simulink model "modeloSimulinkSimscapeHisteresisDeadTime"  (R2025b)
settings: Solver=FixedStepAuto  StartTime=0.0  StopTime=0.04  FixedStep=1e-7  RelTol=1e-3
undefined symbols (not defined in the file): alpha
libraries: fl_lib x50, nesl_utility x26, ee_lib x12, spsTriangleGeneratorLib x6
settings Model: Creator=rkhga  LastModifiedBy=daniel
settings SolverCC: EnableFixedStepZeroCrossing=on

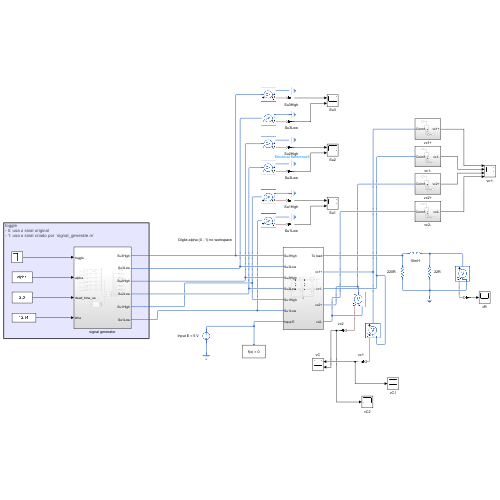
[thumbnail: Simulink's stored preview of the top-level diagram]
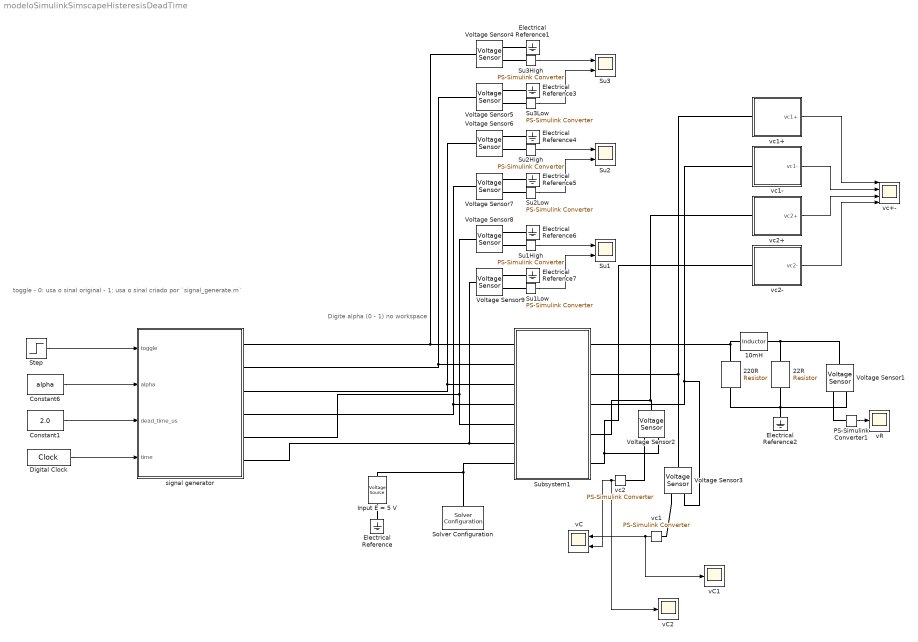
== system modeloSimulinkSimscapeHisteresisDeadTime ==
  note: toggle
      | - 0: usa o sinal original
      | - 1: usa o sinal criado por `signal_generate.m`
  note: Digite alpha (0 - 1) no workspace
  10mH : ee_lib/Passive/Inductor  l=10e-3 H  enable_L_tol=ee.enum.toleranceApplication.none  L_tol=20  tol_distribution=ee.enum.toleranceDistribution.uniform  nSigma=4  r=0 Ohm  g=1e-9 1/Ohm  enable_operating_limits=ee.enum.enable.no  operating_limit_action=ee.enum.passive.reportOpLim.warn  max_working_current=1 A  power_rating=1 W  i_L_specify=off  i_L_priority=High  i_L=0 A  i_L_nominal_specify=off  i_L_nominal_value=1  i_L_nominal_unit=A
  220R : ee_lib/Passive/Resistor  R=220 Ohm  enable_R_tol=ee.enum.toleranceApplication.none  R_tol=5  tol_distribution=ee.enum.toleranceDistribution.uniform  nSigma=4  enable_operating_limits=ee.enum.enable.no  operating_limit_action=ee.enum.passive.reportOpLim.warn  power_rating=1 W  max_working_voltage=100 V  noise_mode=ee.enum.sources.noise.Disabled  Tdevice=25 degC  sample_time=1e-3 s  repeatability=ee.enum.ic.repeatability.notRepeatable  user_seed=0  auto_seed=418932850  power_derating_T1=70 degC  power_derating_T2=155 degC  operating_temperature_range_vec=[-50, 150] degC  alpha=3.93e-3 1/K  Tmeas=25 degC  thermal_mass=100 J/K  temperature_specify=off  temperature_priority=High  temperature=298.15 K  temperature_nominal_specify=off  temperature_nominal_value=1  temperature_nominal_unit=K
  22R : ee_lib/Passive/Resistor  R=22 Ohm  enable_R_tol=ee.enum.toleranceApplication.none  R_tol=5  tol_distribution=ee.enum.toleranceDistribution.uniform  nSigma=4  enable_operating_limits=ee.enum.enable.no  operating_limit_action=ee.enum.passive.reportOpLim.warn  power_rating=1 W  max_working_voltage=100 V  noise_mode=ee.enum.sources.noise.Disabled  Tdevice=25 degC  sample_time=1e-3 s  repeatability=ee.enum.ic.repeatability.notRepeatable  user_seed=0  auto_seed=3890346746  power_derating_T1=70 degC  power_derating_T2=155 degC  operating_temperature_range_vec=[-50, 150] degC  alpha=3.93e-3 1/K  Tmeas=25 degC  thermal_mass=100 J/K  temperature_specify=off  temperature_priority=High  temperature=298.15 K  temperature_nominal_specify=off  temperature_nominal_value=1  temperature_nominal_unit=K
  Constant1 : Constant  Value=2.0
  Constant6 : Constant  Value=alpha
  Digital Clock : DigitalClock  SampleTime=1e-7
  Electrical Reference{,1..7} (8 alike) : fl_lib/Electrical/Electrical Elements/Electrical Reference
  Input E = 5 V : ee_lib/Sources/Voltage Source  dc_voltage=5 V  ac_voltage=0 V  ac_shift=0 rad  ac_frequency=60 Hz  noise_mode=ee.enum.sources.noise.Disabled  PSD=0 V^2/Hz  sample_time=1e-3 s  repeatability=ee.enum.sources.repeatability.NotRepeatable  user_seed=0  auto_seed=3499211588  i_specify=off  i_priority=None  i=0 A  i_nominal_specify=off  i_nominal_value=1  i_nominal_unit=A  v_specify=off  v_priority=None  v=0 V  v_nominal_specify=off  v_nominal_value=1  v_nominal_unit=V
  PS-Simulink Converter1 : nesl_utility/PS-Simulink Converter  PhysicalDomain=network_engine_domain  SubClassName=ps_output  LeftPortType=input  RightPortType=output  PseudoPeriodic=off  Frequencies=[]  VectorFormat=inherit  Unit=inherit  AffineConversion=off
  Solver Configuration : nesl_utility/Solver Configuration  PhysicalDomain=network_engine_domain  SubClassName=solver  LeftPortType=input  RightPortType=generic  Tones=[]  Harmonics=[]  SimulateNoise=off  Profile=off  UseLocalSampling=off  EnableSwitchedLinearOptims=on  FrequencyDomain=off  UseCCode=off  RelTol=0.001  AbsTol=0.001  MinStep=1e-09  ToWorkspace=off  RevertToSquareIcSolve=off  NumHomotopyIterations=100  PhasorMode=off  PhasorModeNumHarmonics=1  ConsistencySolver=NEWTON_XTOL_AFTER_FTOL  IndexReductionMethod=DerivativeReplacement  DoDC=off  ResidualTolerance=1e-09  ConsistencyTolSource=GLOBAL  ConsistencyAbsTol=0.001  ConsistencyRelTol=0.001  ConsistencyTolFactor=0.001  UseLocalSolver=off  LocalSolverChoice=NE_TRAPEZOIDAL_ADVANCER  ResolveIndetEquations=on  FunctionEvalNumThread=1  LocalSolverSampleTime=0.000001  DoFixedCost=off  MaxNonlinIter=3  MaxModeIter=2  ComputeImpulses=off  ImpulseIterations=2  LinearAlgebra=auto  LinearAlgebraNumThread=0  EquationFormulation=NE_TIME_EF  DelaysMemoryBudget=1024  AutomaticFiltering=on  FilteringTimeConstant=0.001  PartitionStorageMethod=AS_NEEDED  PartitionMemoryBudget=1024  PartitionMethod=ROBUST  MultibodyUseLocalSolver=off  MultibodyLocalSolverChoice=ODE1  MultibodyLocalSolverSampleTime=0.001
  Step : Step  Time=0  Before=1  After=0  SampleTime=0
  Su1 : Scope  NumInputPorts=2
      settings: ActiveDisplayYMinimum=0.99850460772373162  ActiveDisplayYMaximum=1.0003414939639432  DataLoggingVariableName=ScopeData3
  Su1High : nesl_utility/PS-Simulink Converter  PhysicalDomain=network_engine_domain  SubClassName=ps_output  LeftPortType=input  RightPortType=output  PseudoPeriodic=off  Frequencies=[]  VectorFormat=inherit  Unit=inherit  AffineConversion=off
  Su1Low : nesl_utility/PS-Simulink Converter  PhysicalDomain=network_engine_domain  SubClassName=ps_output  LeftPortType=input  RightPortType=output  PseudoPeriodic=off  Frequencies=[]  VectorFormat=inherit  Unit=inherit  AffineConversion=off
  Su2 : Scope  NumInputPorts=2
      settings: ActiveDisplayYMinimum=-1.01553  ActiveDisplayYMaximum=1.07216  DataLoggingVariableName=ScopeData2
  Su2High : nesl_utility/PS-Simulink Converter  PhysicalDomain=network_engine_domain  SubClassName=ps_output  LeftPortType=input  RightPortType=output  PseudoPeriodic=off  Frequencies=[]  VectorFormat=inherit  Unit=inherit  AffineConversion=off
  Su2Low : nesl_utility/PS-Simulink Converter  PhysicalDomain=network_engine_domain  SubClassName=ps_output  LeftPortType=input  RightPortType=output  PseudoPeriodic=off  Frequencies=[]  VectorFormat=inherit  Unit=inherit  AffineConversion=off
  Su3 : Scope  NumInputPorts=2
      settings: ActiveDisplayYMinimum=-1.25  ActiveDisplayYMaximum=1.25
  Su3High : nesl_utility/PS-Simulink Converter  PhysicalDomain=network_engine_domain  SubClassName=ps_output  LeftPortType=input  RightPortType=output  PseudoPeriodic=off  Frequencies=[]  VectorFormat=inherit  Unit=inherit  AffineConversion=off
  Su3Low : nesl_utility/PS-Simulink Converter  PhysicalDomain=network_engine_domain  SubClassName=ps_output  LeftPortType=input  RightPortType=output  PseudoPeriodic=off  Frequencies=[]  VectorFormat=inherit  Unit=inherit  AffineConversion=off
  Subsystem1 : Subsystem
  Voltage Sensor{1..9} (9 alike) : fl_lib/Electrical/Electrical Sensors/Voltage Sensor
  signal generator : Subsystem
      settings: PortSchema="{\"entries\":[{\"content\":{\"sides\":[{\"content\":{\"connectorIds\":[\"LConn1\",\"LConn2\",\"LConn3\",\"LConn4\",\"LConn5\",\"LConn6\"]},\"type\":\"ConnectorPlacement.EquallySpacedRectSide\",\"uuid\":\"aa1a153a-1645-4c3d-b48e-03759f31f217\"},{\"content\":{\"connectorIds\":[\"In1\",\"In2\",\"In3\",\"In4\"],\"side\":\"RIGHT\"},\"type\":\"ConnectorPlacement.EquallySpacedRectSide\",\"uuid\":\"be438c4b-dc66-4eaf-bb53-25e90e68573c\"},{\"content\":{\"side\":\"TOP\"},\"type\":\"ConnectorPlacement.EquallySpacedRectSide\",\"uuid\":\"4362158f-9cc4-444f-8c13-d432f498cf5b\"}]},\"type\":\"ConnectorPlacement.EquallySpacedConnector\",\"uuid\":\"f810cfc3-0b98-45ae-8d35-8e9d04ff1bd5\"}],\"packageUris\":[\"http://schema.mathworks.com/mf0/Connector/R2020b\"],\"version\":\"1.0\"}"
  vC : Scope  NumInputPorts=2
      settings: ActiveDisplayYMinimum=-0.84659912811996252  ActiveDisplayYMaximum=6.9513683577501517
  vC1 : Scope
      settings: ActiveDisplayYMinimum=1.5127533601392706  ActiveDisplayYMaximum=1.8347191591870249  DataLoggingVariableName=ScopeData4
  vC2 : Scope
      settings: ActiveDisplayYMinimum=3.0808662411635424  ActiveDisplayYMaximum=3.5294915136441256  DataLoggingVariableName=ScopeData5
  vR : Scope
      settings: ActiveDisplayYMinimum=0.27238883407399678  ActiveDisplayYMaximum=0.38136658735243295
  vc+- : Scope  NumInputPorts=4
      settings: ActiveDisplayYMinimum=-18.52788  ActiveDisplayYMaximum=9.39765
  vc1 : nesl_utility/PS-Simulink Converter  PhysicalDomain=network_engine_domain  SubClassName=ps_output  LeftPortType=input  RightPortType=output  PseudoPeriodic=off  Frequencies=[]  VectorFormat=inherit  Unit=inherit  AffineConversion=off
  vc1+ : Subsystem
  vc1- : Subsystem
  vc2 : nesl_utility/PS-Simulink Converter  PhysicalDomain=network_engine_domain  SubClassName=ps_output  LeftPortType=input  RightPortType=output  PseudoPeriodic=off  Frequencies=[]  VectorFormat=inherit  Unit=inherit  AffineConversion=off
  vc2+ : Subsystem
  vc2- : Subsystem
  wires:
  PS-Simulink Converter1/1 -> vR/1
  vc1/1 -> vC1/1, vC/1
  Su3High/1 -> Su3/1
  Su3Low/1 -> Su3/2
  Su2High/1 -> Su2/1
  Su2Low/1 -> Su2/2
  Su1High/1 -> Su1/1
  Su1Low/1 -> Su1/2
  vc2/1 -> vC2/1, vC/2
  vc2+/1(vc2+) -> vc+-/3
  vc1-/1(vc1-) -> vc+-/2
  vc2-/1(vc2-) -> vc+-/4
  vc1+/1(vc1+) -> vc+-/1
  Step/1 -> signal generator/1(toggle)
  Constant6/1 -> signal generator/2(alpha)
  Digital Clock/1 -> signal generator/4(time)
  Constant1/1 -> signal generator/3(dead_time_us)
  connections:
  Electrical Reference/LConn1 -- Input E = 5 V/RConn1
  Subsystem1/LConn7 -- Solver Configuration/RConn1 -- Input E = 5 V/LConn1
  22R/RConn1 -- 220R/RConn1 -- Electrical Reference2/LConn1 -- Voltage Sensor1/RConn2
  Voltage Sensor1/LConn1 -- 10mH/RConn1 -- 22R/LConn1
  Voltage Sensor1/RConn1 -- PS-Simulink Converter1/LConn1
  220R/LConn1 -- 10mH/LConn1 -- Subsystem1/RConn1
  Subsystem1/LConn1 -- Voltage Sensor4/LConn1 -- signal generator/LConn1
  Subsystem1/LConn2 -- Voltage Sensor5/LConn1 -- signal generator/LConn2
  Subsystem1/LConn3 -- Voltage Sensor6/LConn1 -- signal generator/LConn3
  signal generator/LConn4 -- Voltage Sensor7/LConn1 -- Subsystem1/LConn4
  Subsystem1/LConn5 -- signal generator/LConn5 -- Voltage Sensor8/LConn1
  signal generator/LConn6 -- Voltage Sensor9/LConn1 -- Subsystem1/LConn6
  Subsystem1/RConn4 -- vc2+/LConn1 -- Voltage Sensor2/LConn1
  Voltage Sensor2/RConn2 -- vc2-/LConn1 -- Subsystem1/RConn5
  Voltage Sensor3/RConn1 -- vc1/LConn1
  Subsystem1/RConn2 -- vc1+/LConn1 -- Voltage Sensor3/LConn1
  Subsystem1/RConn3 -- vc1-/LConn1 -- Voltage Sensor3/RConn2
  Electrical Reference1/LConn1 -- Voltage Sensor4/RConn2
  Voltage Sensor5/RConn2 -- Electrical Reference3/LConn1
  Voltage Sensor4/RConn1 -- Su3High/LConn1
  Su3Low/LConn1 -- Voltage Sensor5/RConn1
  Voltage Sensor6/RConn1 -- Su2High/LConn1
  Electrical Reference4/LConn1 -- Voltage Sensor6/RConn2
  Su2Low/LConn1 -- Voltage Sensor7/RConn1
  Voltage Sensor7/RConn2 -- Electrical Reference5/LConn1
  Voltage Sensor8/RConn1 -- Su1High/LConn1
  Voltage Sensor9/RConn2 -- Electrical Reference7/LConn1
  Electrical Reference6/LConn1 -- Voltage Sensor8/RConn2
  Su1Low/LConn1 -- Voltage Sensor9/RConn1
  Voltage Sensor2/RConn1 -- vc2/LConn1

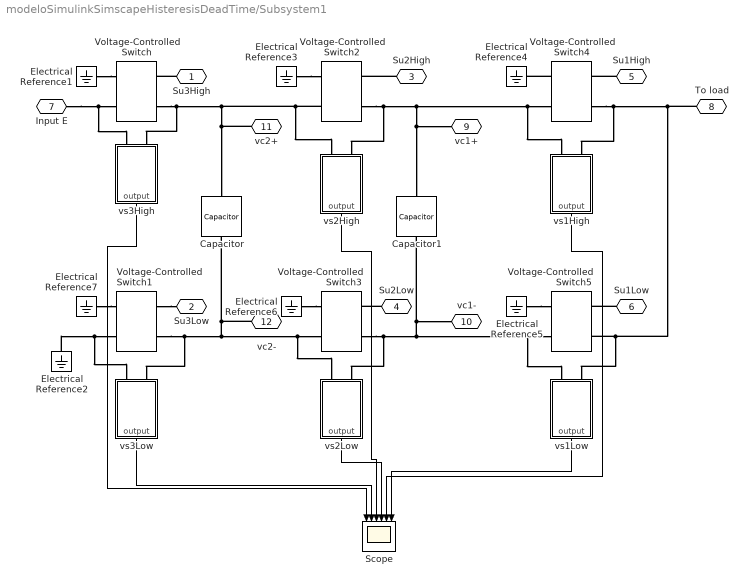
== system modeloSimulinkSimscapeHisteresisDeadTime/Subsystem1 ==
  Capacitor : ee_lib/Passive/Capacitor  cap_option=ee.enum.passive.capacitor.capOption.const  c=2.1e-6 F  Cvec=[1e-05, 1e-06] F  Vvec=[0, 10] V  CV_table_symmetry=ee.enum.passive.capacitor.tableSymmetry.yes  f_vec=[1, 10] kHz  DFext_vec=[.8, 1.2]  enable_C_tol=ee.enum.toleranceApplication.none  averaging_period=0 s  C_tol=5  tol_distribution=ee.enum.toleranceDistribution.uniform  nSigma=4  r=0 Ohm  g=0 1/Ohm  enable_operating_limits=ee.enum.enable.no  operating_limit_action=ee.enum.passive.reportOpLim.warn  max_working_voltage_range=[-25, 25] V  power_rating=1 W  maxTemperature=85 degC  thermalEnable=false  thermalMass=1 J/K  i_specify=off  i_priority=None  i=0 A  i_nominal_specify=off  i_nominal_value=1  i_nominal_unit=A  v_specify=off  v_priority=None  v=0 V  v_nominal_specify=off  v_nominal_value=1  v_nominal_unit=V  vc_specify=off  vc_priority=High  vc=0 V  vc_nominal_specify=off  vc_nominal_value=1  vc_nominal_unit=V  T_specify=off  T_priority=None  T=298.15 K  T_nominal_specify=off  T_nominal_value=1  T_nominal_unit=K
  Capacitor1 : ee_lib/Passive/Capacitor  cap_option=ee.enum.passive.capacitor.capOption.const  c=2.1e-6 F  Cvec=[1e-05, 1e-06] F  Vvec=[0, 10] V  CV_table_symmetry=ee.enum.passive.capacitor.tableSymmetry.yes  f_vec=[1, 10] kHz  DFext_vec=[.8, 1.2]  enable_C_tol=ee.enum.toleranceApplication.none  averaging_period=0 s  C_tol=5  tol_distribution=ee.enum.toleranceDistribution.uniform  nSigma=4  r=0 Ohm  g=0 1/Ohm  enable_operating_limits=ee.enum.enable.no  operating_limit_action=ee.enum.passive.reportOpLim.warn  max_working_voltage_range=[-25, 25] V  power_rating=1 W  maxTemperature=85 degC  thermalEnable=false  thermalMass=1 J/K  i_specify=off  i_priority=None  i=0 A  i_nominal_specify=off  i_nominal_value=1  i_nominal_unit=A  v_specify=off  v_priority=None  v=0 V  v_nominal_specify=off  v_nominal_value=1  v_nominal_unit=V  vc_specify=off  vc_priority=High  vc=0 V  vc_nominal_specify=off  vc_nominal_value=1  vc_nominal_unit=V  T_specify=off  T_priority=None  T=298.15 K  T_nominal_specify=off  T_nominal_value=1  T_nominal_unit=K
  Electrical Reference{1..7} (7 alike) : fl_lib/Electrical/Electrical Elements/Electrical Reference
  Scope : Scope  NumInputPorts=6
      settings: ActiveDisplayYMinimum=-8.8853464798149755  ActiveDisplayYMaximum=25.227625908816535  DataLoggingVariableName=ScopeData2
  Voltage-Controlled Switch{,1..5} (6 alike) : ee_lib/Additional Components/SPICE Passives/Voltage-Controlled Switch  SWITCH_model=ee.enum.switches.switchModelVoltage.transition  VON=1 V  VOFF=0 V  VT=0 V  VH=0 V  RON=1e-12 Ohm  ROFF_res=1e6 Ohm  Roff_gmin=ee.enum.switches.offResistance.no  ROFF=1e12 Ohm  TD=0 s
      settings: InternalSimscapePortConfiguration="{\"Bottom\":[],\"Left\":[{\"id\":\"p1\",\"label\":\"1+\",\"type\":\"foundation.electrical.electrical\"},{\"id\":\"p2\",\"label\":\"2+\",\"type\":\"foundation.electrical.electrical\"}],\"Right\":[{\"id\":\"n1\",\"label\":\"1-\",\"type\":\"foundation.electrical.electrical\"},{\"id\":\"n2\",\"label\":\"2-\",\"type\":\"foundation.electrical.electrical\"}],\"Top\":[]}"
  vs1High : Subsystem
  vs1Low : Subsystem
  vs2High : Subsystem
  vs2Low : Subsystem
  vs3High : Subsystem
  vs3Low : Subsystem
  Su3High : PMIOPort  Side=Left
  Su3Low : PMIOPort  Port=2  Side=Left
  Su2High : PMIOPort  Port=3  Side=Left
  Su2Low : PMIOPort  Port=4  Side=Left
  Su1High : PMIOPort  Port=5  Side=Left
  Su1Low : PMIOPort  Port=6  Side=Left
  Input E : PMIOPort  Port=7  Side=Left
  To load : PMIOPort  Port=8  Side=Right
  vc1+ : PMIOPort  Port=9  Side=Right
  vc1- : PMIOPort  Port=10  Side=Right
  vc2+ : PMIOPort  Port=11  Side=Right
  vc2- : PMIOPort  Port=12  Side=Right
  wires:
  vs2Low/1(output) -> Scope/4
  vs1Low/1(output) -> Scope/6
  vs3Low/1(output) -> Scope/2
  vs2High/1(output) -> Scope/3
  vs1High/1(output) -> Scope/5
  vs3High/1(output) -> Scope/1
  connections:
  Su2Low/RConn1 -- Voltage-Controlled Switch3/LConn1
  Voltage-Controlled Switch2/LConn2 -- vs2High/LConn2 -- vc1+/RConn1 -- Capacitor1/LConn1 -- vs1High/LConn1 -- Voltage-Controlled Switch4/RConn2
  Input E/RConn1 -- vs3High/LConn1 -- Voltage-Controlled Switch/RConn2
  Voltage-Controlled Switch/LConn2 -- vs2High/LConn1 -- Voltage-Controlled Switch2/RConn2 -- vc2+/RConn1 -- Capacitor/LConn1 -- vs3High/LConn2
  Voltage-Controlled Switch3/LConn2 -- vs2Low/LConn2 -- Capacitor1/RConn1 -- vc1-/RConn1 -- vs1Low/LConn1 -- Voltage-Controlled Switch5/RConn2
  Voltage-Controlled Switch1/LConn2 -- vs3Low/LConn2 -- Capacitor/RConn1 -- vc2-/RConn1 -- vs2Low/LConn1 -- Voltage-Controlled Switch3/RConn2
  Voltage-Controlled Switch4/LConn2 -- vs1High/LConn2 -- To load/RConn1 -- vs1Low/LConn2 -- Voltage-Controlled Switch5/LConn2
  Electrical Reference2/LConn1 -- vs3Low/LConn1 -- Voltage-Controlled Switch1/RConn2
  Voltage-Controlled Switch1/LConn1 -- Su3Low/RConn1
  Su1High/RConn1 -- Voltage-Controlled Switch4/LConn1
  Su2High/RConn1 -- Voltage-Controlled Switch2/LConn1
  Su3High/RConn1 -- Voltage-Controlled Switch/LConn1
  Electrical Reference1/LConn1 -- Voltage-Controlled Switch/RConn1
  Electrical Reference3/LConn1 -- Voltage-Controlled Switch2/RConn1
  Electrical Reference5/LConn1 -- Voltage-Controlled Switch5/RConn1
  Electrical Reference6/LConn1 -- Voltage-Controlled Switch3/RConn1
  Su1Low/RConn1 -- Voltage-Controlled Switch5/LConn1
  Electrical Reference7/LConn1 -- Voltage-Controlled Switch1/RConn1
  Voltage-Controlled Switch4/RConn1 -- Electrical Reference4/LConn1

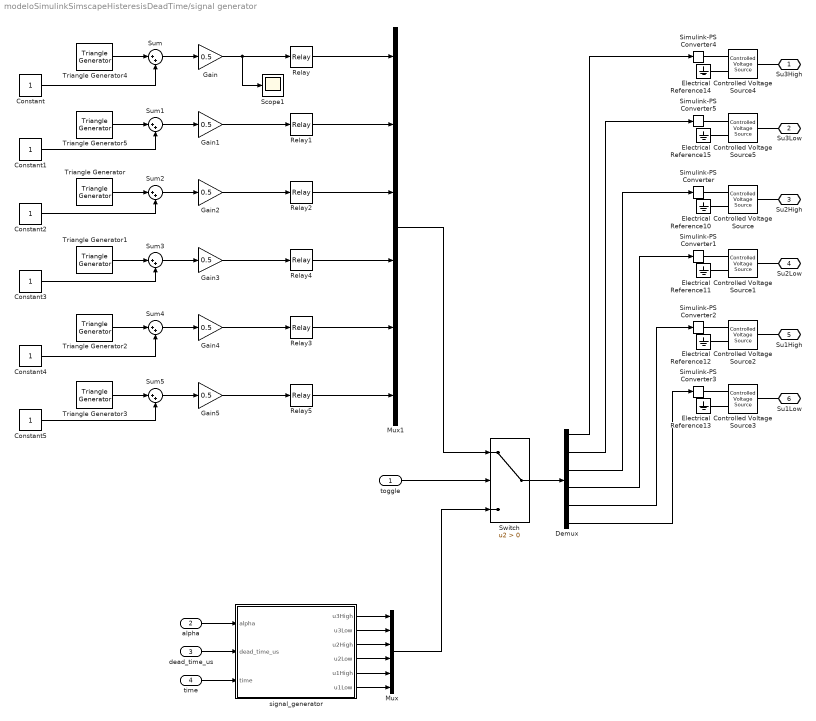
== system modeloSimulinkSimscapeHisteresisDeadTime/signal generator ==
  toggle : Inport
  alpha : Inport  Port=2
  dead_time_us : Inport  Port=3
  time : Inport  Port=4
  Constant{,1..5} (6 alike) : Constant
  Controlled Voltage Source{,1..5} (6 alike) : fl_lib/Electrical/Electrical Sources/Controlled Voltage Source
  Demux : Demux  Outputs=6
  Electrical Reference{10..15} (6 alike) : fl_lib/Electrical/Electrical Elements/Electrical Reference
  Gain{,1..5} (6 alike) : Gain  Gain=0.5
  Mux : Mux  Inputs=6
  Mux1 : Mux  Inputs=6
  Relay : Relay  OnSwitchValue=alpha  OffSwitchValue=alpha - 2/141  OnOutputValue=-1  OffOutputValue=1
  Relay1 : Relay  OnSwitchValue=alpha + 2/141  OffSwitchValue=alpha  OnOutputValue=+1  OffOutputValue=-1
  Relay2 : Relay  OnSwitchValue=alpha  OffSwitchValue=alpha - 2/141  OnOutputValue=-1  OffOutputValue=1
  Relay3 : Relay  OnSwitchValue=alpha  OffSwitchValue=alpha - 2/141  OnOutputValue=-1  OffOutputValue=1
  Relay4 : Relay  OnSwitchValue=alpha + 2/141  OffSwitchValue=alpha  OnOutputValue=+1  OffOutputValue=-1
  Relay5 : Relay  OnSwitchValue=alpha + 2/141  OffSwitchValue=alpha  OnOutputValue=+1  OffOutputValue=-1
  Scope1 : Scope
      settings: ActiveDisplayYMinimum=-0.04742  ActiveDisplayYMaximum=1.07583  DataLoggingVariableName=ScopeData2
  Simulink-PS Converter{,1..5} (6 alike) : nesl_utility/Simulink-PS Converter  PhysicalDomain=network_engine_domain  SubClassName=ps_input  LeftPortType=input  RightPortType=output  PseudoPeriodic=off  Frequencies=[]  NoiseDistribution=none  NoiseParameters=[]  Unit=1  AffineConversion=off  FilteringAndDerivatives=provide  SimscapeFilterOrder=1  InputFilterTimeConstant=0.001  UdotUserProvided=0
  Sum{,1..5} (6 alike) : Sum  Inputs=|++
  Switch : Switch  Criteria=u2 > Threshold  SaturateOnIntegerOverflow=off  InputSameDT=off
  Triangle Generator : spsTriangleGeneratorLib/Triangle Generator  Freq=1/(282e-6)  Phase=-120  Ts=0
  Triangle Generator1 : spsTriangleGeneratorLib/Triangle Generator  Freq=1/(282e-6)  Phase=-120  Ts=0
  Triangle Generator2 : spsTriangleGeneratorLib/Triangle Generator  Freq=1/(282e-6)  Phase=-240  Ts=0
  Triangle Generator3 : spsTriangleGeneratorLib/Triangle Generator  Freq=1/(282e-6)  Phase=-240  Ts=0
  Triangle Generator4 : spsTriangleGeneratorLib/Triangle Generator  Freq=1/(282e-6)  Phase=0  Ts=0
  Triangle Generator5 : spsTriangleGeneratorLib/Triangle Generator  Freq=1/(282e-6)  Phase=0  Ts=0
  signal_generator : Subsystem
  Su3High : PMIOPort  Side=Left
  Su3Low : PMIOPort  Port=2  Side=Left
  Su2High : PMIOPort  Port=3  Side=Left
  Su2Low : PMIOPort  Port=4  Side=Left
  Su1High : PMIOPort  Port=5  Side=Left
  Su1Low : PMIOPort  Port=6  Side=Left
  wires:
  Gain/1 -> Scope1/1, Relay/1
  Gain1/1 -> Relay1/1
  Gain2/1 -> Relay2/1
  Gain3/1 -> Relay4/1
  Gain4/1 -> Relay3/1
  Gain5/1 -> Relay5/1
  Constant/1 -> Sum/2
  Constant1/1 -> Sum1/2
  Constant2/1 -> Sum2/2
  Constant3/1 -> Sum3/2
  Constant4/1 -> Sum4/2
  Constant5/1 -> Sum5/2
  Triangle Generator3/1 -> Sum5/1
  Sum5/1 -> Gain5/1
  Triangle Generator2/1 -> Sum4/1
  Sum4/1 -> Gain4/1
  Triangle Generator1/1 -> Sum3/1
  Sum3/1 -> Gain3/1
  Triangle Generator/1 -> Sum2/1
  Sum2/1 -> Gain2/1
  Triangle Generator5/1 -> Sum1/1
  Sum1/1 -> Gain1/1
  Triangle Generator4/1 -> Sum/1
  Sum/1 -> Gain/1
  time/1 -> signal_generator/3(time)
  alpha/1 -> signal_generator/1(alpha)
  signal_generator/6(u1Low) -> Mux/6
  signal_generator/5(u1High) -> Mux/5
  signal_generator/4(u2Low) -> Mux/4
  signal_generator/3(u2High) -> Mux/3
  signal_generator/2(u3Low) -> Mux/2
  signal_generator/1(u3High) -> Mux/1
  Mux/1 -> Switch/3
  Switch/1 -> Demux/1
  Relay4/1 -> Mux1/4
  Relay2/1 -> Mux1/3
  Relay3/1 -> Mux1/5
  Relay1/1 -> Mux1/2
  Relay5/1 -> Mux1/6
  Relay/1 -> Mux1/1
  toggle/1 -> Switch/2
  Demux/6 -> Simulink-PS Converter3/1
  Demux/5 -> Simulink-PS Converter2/1
  Demux/4 -> Simulink-PS Converter1/1
  Demux/3 -> Simulink-PS Converter/1
  Demux/2 -> Simulink-PS Converter5/1
  Demux/1 -> Simulink-PS Converter4/1
  dead_time_us/1 -> signal_generator/2(dead_time_us)
  Mux1/1 -> Switch/1
  connections:
  Electrical Reference12/LConn1 -- Controlled Voltage Source2/RConn2
  Electrical Reference10/LConn1 -- Controlled Voltage Source/RConn2
  Electrical Reference13/LConn1 -- Controlled Voltage Source3/RConn2
  Simulink-PS Converter3/RConn1 -- Controlled Voltage Source3/RConn1
  Controlled Voltage Source/LConn1 -- Su2High/RConn1
  Simulink-PS Converter5/RConn1 -- Controlled Voltage Source5/RConn1
  Simulink-PS Converter1/RConn1 -- Controlled Voltage Source1/RConn1
  Controlled Voltage Source5/LConn1 -- Su3Low/RConn1
  Simulink-PS Converter2/RConn1 -- Controlled Voltage Source2/RConn1
  Electrical Reference11/LConn1 -- Controlled Voltage Source1/RConn2
  Controlled Voltage Source1/LConn1 -- Su2Low/RConn1
  Electrical Reference15/LConn1 -- Controlled Voltage Source5/RConn2
  Controlled Voltage Source4/LConn1 -- Su3High/RConn1
  Simulink-PS Converter/RConn1 -- Controlled Voltage Source/RConn1
  Controlled Voltage Source3/LConn1 -- Su1Low/RConn1
  Controlled Voltage Source2/LConn1 -- Su1High/RConn1
  Simulink-PS Converter4/RConn1 -- Controlled Voltage Source4/RConn1
  Electrical Reference14/LConn1 -- Controlled Voltage Source4/RConn2

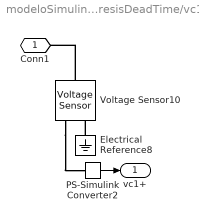
== system modeloSimulinkSimscapeHisteresisDeadTime/vc1+ ==
  Electrical Reference8 : fl_lib/Electrical/Electrical Elements/Electrical Reference
  PS-Simulink Converter2 : nesl_utility/PS-Simulink Converter  PhysicalDomain=network_engine_domain  SubClassName=ps_output  LeftPortType=input  RightPortType=output  PseudoPeriodic=off  Frequencies=[]  VectorFormat=inherit  Unit=inherit  AffineConversion=off
  Voltage Sensor10 : fl_lib/Electrical/Electrical Sensors/Voltage Sensor
  Conn1 : PMIOPort  Side=Left
  vc1+ : Outport
  wires:
  PS-Simulink Converter2/1 -> vc1+/1
  connections:
  Electrical Reference8/LConn1 -- Voltage Sensor10/RConn2
  Voltage Sensor10/LConn1 -- Conn1/RConn1
  Voltage Sensor10/RConn1 -- PS-Simulink Converter2/LConn1

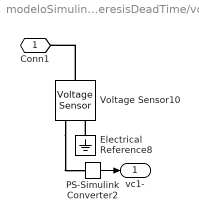
== system modeloSimulinkSimscapeHisteresisDeadTime/vc1- ==
  Electrical Reference8 : fl_lib/Electrical/Electrical Elements/Electrical Reference
  PS-Simulink Converter2 : nesl_utility/PS-Simulink Converter  PhysicalDomain=network_engine_domain  SubClassName=ps_output  LeftPortType=input  RightPortType=output  PseudoPeriodic=off  Frequencies=[]  VectorFormat=inherit  Unit=inherit  AffineConversion=off
  Voltage Sensor10 : fl_lib/Electrical/Electrical Sensors/Voltage Sensor
  Conn1 : PMIOPort  Side=Left
  vc1- : Outport
  wires:
  PS-Simulink Converter2/1 -> vc1-/1
  connections:
  Voltage Sensor10/RConn1 -- PS-Simulink Converter2/LConn1
  Voltage Sensor10/LConn1 -- Conn1/RConn1
  Electrical Reference8/LConn1 -- Voltage Sensor10/RConn2

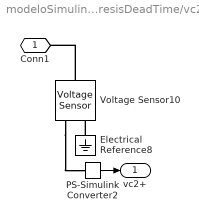
== system modeloSimulinkSimscapeHisteresisDeadTime/vc2+ ==
  Electrical Reference8 : fl_lib/Electrical/Electrical Elements/Electrical Reference
  PS-Simulink Converter2 : nesl_utility/PS-Simulink Converter  PhysicalDomain=network_engine_domain  SubClassName=ps_output  LeftPortType=input  RightPortType=output  PseudoPeriodic=off  Frequencies=[]  VectorFormat=inherit  Unit=inherit  AffineConversion=off
  Voltage Sensor10 : fl_lib/Electrical/Electrical Sensors/Voltage Sensor
  Conn1 : PMIOPort  Side=Left
  vc2+ : Outport
  wires:
  PS-Simulink Converter2/1 -> vc2+/1
  connections:
  Electrical Reference8/LConn1 -- Voltage Sensor10/RConn2
  Voltage Sensor10/LConn1 -- Conn1/RConn1
  Voltage Sensor10/RConn1 -- PS-Simulink Converter2/LConn1

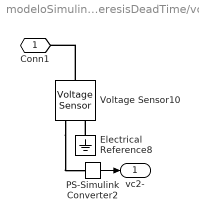
== system modeloSimulinkSimscapeHisteresisDeadTime/vc2- ==
  Electrical Reference8 : fl_lib/Electrical/Electrical Elements/Electrical Reference
  PS-Simulink Converter2 : nesl_utility/PS-Simulink Converter  PhysicalDomain=network_engine_domain  SubClassName=ps_output  LeftPortType=input  RightPortType=output  PseudoPeriodic=off  Frequencies=[]  VectorFormat=inherit  Unit=inherit  AffineConversion=off
  Voltage Sensor10 : fl_lib/Electrical/Electrical Sensors/Voltage Sensor
  Conn1 : PMIOPort  Side=Left
  vc2- : Outport
  wires:
  PS-Simulink Converter2/1 -> vc2-/1
  connections:
  Voltage Sensor10/RConn1 -- PS-Simulink Converter2/LConn1
  Voltage Sensor10/LConn1 -- Conn1/RConn1
  Electrical Reference8/LConn1 -- Voltage Sensor10/RConn2

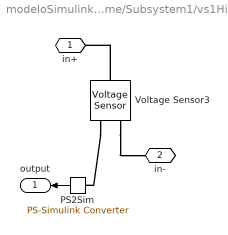
== system modeloSimulinkSimscapeHisteresisDeadTime/Subsystem1/vs1High ==
  PS2Sim : nesl_utility/PS-Simulink Converter  PhysicalDomain=network_engine_domain  SubClassName=ps_output  LeftPortType=input  RightPortType=output  PseudoPeriodic=off  Frequencies=[]  VectorFormat=inherit  Unit=inherit  AffineConversion=off
  Voltage Sensor3 : fl_lib/Electrical/Electrical Sensors/Voltage Sensor
  in+ : PMIOPort  Side=Left
  in- : PMIOPort  Port=2  Side=Left
  output : Outport
  wires:
  PS2Sim/1 -> output/1
  connections:
  Voltage Sensor3/RConn1 -- PS2Sim/LConn1
  Voltage Sensor3/RConn2 -- in-/RConn1
  Voltage Sensor3/LConn1 -- in+/RConn1

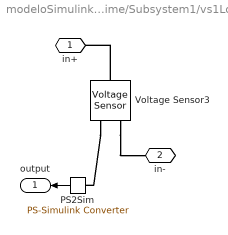
== system modeloSimulinkSimscapeHisteresisDeadTime/Subsystem1/vs1Low ==
  PS2Sim : nesl_utility/PS-Simulink Converter  PhysicalDomain=network_engine_domain  SubClassName=ps_output  LeftPortType=input  RightPortType=output  PseudoPeriodic=off  Frequencies=[]  VectorFormat=inherit  Unit=inherit  AffineConversion=off
  Voltage Sensor3 : fl_lib/Electrical/Electrical Sensors/Voltage Sensor
  in+ : PMIOPort  Side=Left
  in- : PMIOPort  Port=2  Side=Left
  output : Outport
  wires:
  PS2Sim/1 -> output/1
  connections:
  Voltage Sensor3/LConn1 -- in+/RConn1
  Voltage Sensor3/RConn2 -- in-/RConn1
  Voltage Sensor3/RConn1 -- PS2Sim/LConn1

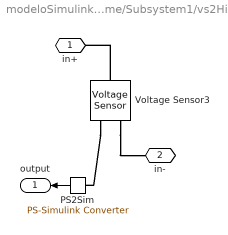
== system modeloSimulinkSimscapeHisteresisDeadTime/Subsystem1/vs2High ==
  PS2Sim : nesl_utility/PS-Simulink Converter  PhysicalDomain=network_engine_domain  SubClassName=ps_output  LeftPortType=input  RightPortType=output  PseudoPeriodic=off  Frequencies=[]  VectorFormat=inherit  Unit=inherit  AffineConversion=off
  Voltage Sensor3 : fl_lib/Electrical/Electrical Sensors/Voltage Sensor
  in+ : PMIOPort  Side=Left
  in- : PMIOPort  Port=2  Side=Left
  output : Outport
  wires:
  PS2Sim/1 -> output/1
  connections:
  Voltage Sensor3/LConn1 -- in+/RConn1
  Voltage Sensor3/RConn2 -- in-/RConn1
  Voltage Sensor3/RConn1 -- PS2Sim/LConn1

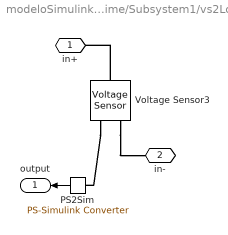
== system modeloSimulinkSimscapeHisteresisDeadTime/Subsystem1/vs2Low ==
  PS2Sim : nesl_utility/PS-Simulink Converter  PhysicalDomain=network_engine_domain  SubClassName=ps_output  LeftPortType=input  RightPortType=output  PseudoPeriodic=off  Frequencies=[]  VectorFormat=inherit  Unit=inherit  AffineConversion=off
  Voltage Sensor3 : fl_lib/Electrical/Electrical Sensors/Voltage Sensor
  in+ : PMIOPort  Side=Left
  in- : PMIOPort  Port=2  Side=Left
  output : Outport
  wires:
  PS2Sim/1 -> output/1
  connections:
  Voltage Sensor3/RConn1 -- PS2Sim/LConn1
  Voltage Sensor3/RConn2 -- in-/RConn1
  Voltage Sensor3/LConn1 -- in+/RConn1

== system modeloSimulinkSimscapeHisteresisDeadTime/Subsystem1/vs3High ==
  PS2Sim : nesl_utility/PS-Simulink Converter  PhysicalDomain=network_engine_domain  SubClassName=ps_output  LeftPortType=input  RightPortType=output  PseudoPeriodic=off  Frequencies=[]  VectorFormat=inherit  Unit=inherit  AffineConversion=off
  Voltage Sensor3 : fl_lib/Electrical/Electrical Sensors/Voltage Sensor
  in+ : PMIOPort  Side=Left
  in- : PMIOPort  Port=2  Side=Left
  output : Outport
  wires:
  PS2Sim/1 -> output/1
  connections:
  Voltage Sensor3/RConn1 -- PS2Sim/LConn1
  Voltage Sensor3/RConn2 -- in-/RConn1
  Voltage Sensor3/LConn1 -- in+/RConn1

== system modeloSimulinkSimscapeHisteresisDeadTime/Subsystem1/vs3Low ==
  PS2Sim : nesl_utility/PS-Simulink Converter  PhysicalDomain=network_engine_domain  SubClassName=ps_output  LeftPortType=input  RightPortType=output  PseudoPeriodic=off  Frequencies=[]  VectorFormat=inherit  Unit=inherit  AffineConversion=off
  Voltage Sensor3 : fl_lib/Electrical/Electrical Sensors/Voltage Sensor
  in+ : PMIOPort  Side=Left
  in- : PMIOPort  Port=2  Side=Left
  output : Outport
  wires:
  PS2Sim/1 -> output/1
  connections:
  Voltage Sensor3/LConn1 -- in+/RConn1
  Voltage Sensor3/RConn2 -- in-/RConn1
  Voltage Sensor3/RConn1 -- PS2Sim/LConn1

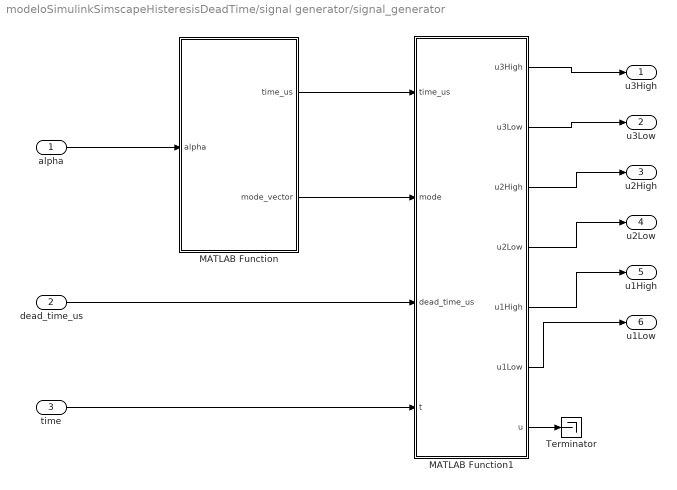
== system modeloSimulinkSimscapeHisteresisDeadTime/signal generator/signal_generator ==
  alpha : Inport
  dead_time_us : Inport  Port=2
  time : Inport  Port=3
  MATLAB Function : MATLAB Function  TreatAsAtomicUnit=on
  MATLAB Function1 : MATLAB Function  TreatAsAtomicUnit=on
  Terminator : Terminator
  u3High : Outport
  u3Low : Outport  Port=2
  u2High : Outport  Port=3
  u2Low : Outport  Port=4
  u1High : Outport  Port=5
  u1Low : Outport  Port=6
  wires:
  MATLAB Function/2(mode_vector) -> MATLAB Function1/2(mode)
  MATLAB Function/1(time_us) -> MATLAB Function1/1(time_us)
  alpha/1 -> MATLAB Function/1(alpha)
  time/1 -> MATLAB Function1/4(t)
  MATLAB Function1/7(u) -> Terminator/1
  MATLAB Function1/1(u3High) -> u3High/1
  MATLAB Function1/2(u3Low) -> u3Low/1
  MATLAB Function1/3(u2High) -> u2High/1
  MATLAB Function1/4(u2Low) -> u2Low/1
  MATLAB Function1/5(u1High) -> u1High/1
  MATLAB Function1/6(u1Low) -> u1Low/1
  dead_time_us/1 -> MATLAB Function1/3(dead_time_us)

== matlab function modeloSimulinkSimscapeHisteresisDeadTime/signal generator/signal_generator/MATLAB Function1 ==
  data: time_us input; u3High output; mode input; dead_time_us input; t input; u3Low output; u2High output; u2Low output; u1High output; u1Low output; u output
function [u3High, u3Low ,u2High, u2Low ,u1High, u1Low, u] = generate_signal(time_us, mode, dead_time_us, t)

    [u3High, u3Low ,u2High, u2Low ,u1High, u1Low, u] = signal_generate(time_us, mode, dead_time_us, t);

== matlab function modeloSimulinkSimscapeHisteresisDeadTime/signal generator/signal_generator/MATLAB Function ==
  data: alpha input; time_us output; mode_vector output
function [time_us, mode_vector] = fcn(alpha)
    [time_us, mode_vector] = signal_create(alpha);
